simulink model "PlantModelOnHardware"  (R2018a)
settings: Solver=VariableStepAuto  StartTime=0.0  StopTime=40  RelTol=1e-3
values from neighbouring files (symbols this model uses):
  K = lqr(A,B,Qc,Rc)    [lqr_controller.m]
undefined symbols (not defined in the file or in its folder): Continuous, HIL, qc_get_step_size, Time
libraries: quarc_library x6, simulink x1, ctrlSharedLib x1
settings Model: Creator=romeo  LastModifiedBy=romeo

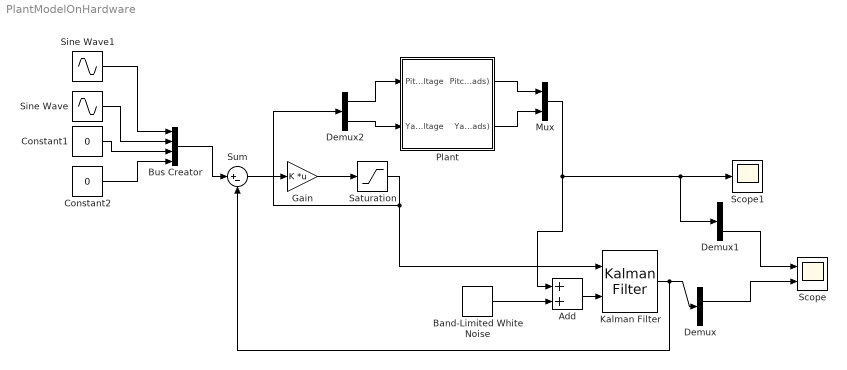
== system PlantModelOnHardware ==
  Add : Sum
  Band-Limited White Noise : simulink/Sources/Band-Limited White Noise  Cov=[0.01]  Ts=0.1  seed=[23341]
  Bus Creator : BusCreator  Inputs=4
  Constant1 : Constant  Value=0
  Constant2 : Constant  Value=0
  Demux : Demux
  Demux1 : Demux  Outputs=2
  Demux2 : Demux  Outputs=2
  Gain : Gain  Gain=K  Multiplication=Matrix(K*u)
  Kalman Filter : ctrlSharedLib/Kalman Filter  TimeDomain=Continuous-Time  UseCurrentEstimator=off  ModelSource=LTI State-Space Variable  ModelSourceVariable=sys  A=0.95  B=1  C=1  D=0  NumberOfStates=1  NumberOfInputs=1  NumberOfOutputs=1  InitialEstimateSource=Dialog  X0=0  P0=10  UseK=off  UseGH=off  NumberOfProcessNoiseInputs=1  G=1  TimeInvariantG=on  H=0  TimeInvariantH=on  Q=0.05  TimeInvariantQ=on  R=1  TimeInvariantR=on  N=0  TimeInvariantN=on  AddInputPort=on  AddEnablePort=off  OutputEstimatedY=off  OutputP=off  Ts=-1
      settings: SourceProductBaseCode=CT
  Mux : Mux  Inputs=2
  Plant : Subsystem
  Saturation : Saturate  UpperLimit=25  LowerLimit=-25
  Scope : Scope  NumInputPorts=2
  Scope1 : Scope
  Sine Wave : Sin  Amplitude=10  SampleTime=0
  Sine Wave1 : Sin  Amplitude=10  SampleTime=0
  Sum : Sum  Inputs=|+-
  wires:
  Saturation/1 -> Demux2/1, Kalman Filter/1
  Mux/1 -> Add/1, Demux1/1, Scope1/1
  Kalman Filter/1 -> Demux/1, Sum/2
  Demux1/2 -> Scope/1
  Demux/2 -> Scope/2
  Add/1 -> Kalman Filter/2
  Band-Limited White Noise/1 -> Add/2
  Sine Wave1/1 -> Bus Creator/1
  Sine Wave/1 -> Bus Creator/2
  Constant1/1 -> Bus Creator/3
  Constant2/1 -> Bus Creator/4
  Bus Creator/1 -> Sum/1
  Sum/1 -> Gain/1
  Gain/1 -> Saturation/1
  Plant/1(Pitch Position (rads)) -> Mux/1
  Plant/2(Yaw Position (rads)) -> Mux/2
  Demux2/1 -> Plant/1(Pitch Voltage)
  Demux2/2 -> Plant/2(Yaw Voltage)

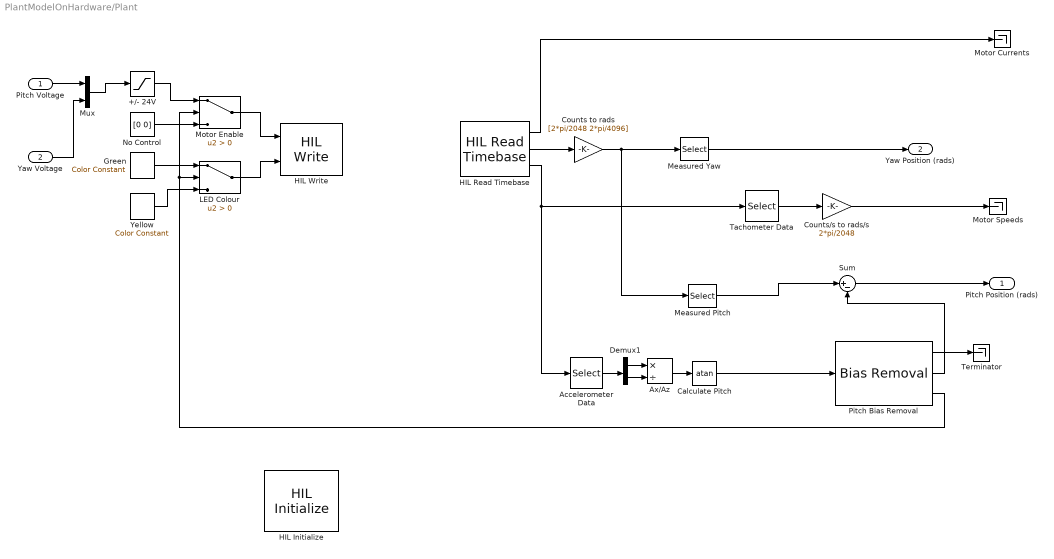
== system PlantModelOnHardware/Plant ==
  Pitch Voltage : Inport
  Yaw Voltage : Inport  Port=2
  +/- 24V : Saturate  UpperLimit=24  LowerLimit=-24
  Accelerometer Data : Selector  InputPortWidth=4  IndexOptions=Index vector (dialog)  Indices=[1 2]  OutputSizes=1
  Ax/Az : Product  Inputs=*/
  Calculate Pitch : Trigonometry  Operator=atan
  Counts to rads : Gain  Gain=[2*pi/2048 2*pi/4096]
  Counts/s to rads/s : Gain  Gain=2*pi/2048
  Demux1 : Demux  Outputs=2
  Green : quarc_library/Sources/Signals/Color Constant  color=[0 1 0]
  HIL Initialize : quarc_library/Data Acquisition/Generic/Configuration/HIL Initialize  Priority=-99  object_name=HIL-1  board_type=quanser_aero_usb  board_number=0  board_options=""  exclusive=off  active=off  hardware_clocks=[0]  clock_modes=[]  initial_clock_frequencies=[]  set_clock_params_at_start=off  set_clock_params_at_switch_in=off  set_clock_frequencies_at_start=off  set_clock_frequencies_at_switch_in=off  analog_input_channels=[0:1]  analog_input_configurations=0  analog_input_maximums=3  analog_input_minimums=-3  set_analog_input_params_at_start=off  set_analog_input_params_at_switch_in=off  analog_output_channels=[0:1]  analog_output_maximums=24  analog_output_minimums=-24  initial_analog_outputs=[0]  final_analog_outputs=[0]  watchdog_analog_outputs=[0]  set_analog_output_params_at_start=off  set_analog_output_params_at_switch_in=off  set_analog_outputs_at_start=on  set_analog_outputs_at_switch_in=off  set_analog_outputs_at_terminate=on  set_analog_outputs_at_switch_out=off  set_analog_outputs_on_watchdog=on  digital_input_channels=[]  digital_output_channels=[0:1]  digital_output_configuration=[]  initial_digital_outputs=[1]  final_digital_outputs=[0]  watchdog_digital_outputs=[0]  set_digital_output_params_at_start=off  set_digital_output_params_at_switch_in=off  set_digital_outputs_at_start=on  set_digital_outputs_at_switch_in=off  set_digital_outputs_at_terminate=on  set_digital_outputs_at_switch_out=off  set_digital_outputs_on_watchdog=on  encoder_channels=[0:3]  quadrature=[4]  encoder_filter_frequency=[]  initial_encoder_counts=[0]  set_encoder_params_at_start=off  set_encoder_params_at_switch_in=off  set_encoder_counts_at_start=on  set_encoder_counts_at_switch_in=off  pwm_channels=[]  pwm_modes=[]  pwm_frequency=[]  pwm_configuration=[]  pwm_alignment=[]  pwm_polarity=[]  pwm_leading_deadband=[]  pwm_trailing_deadband=[]  initial_pwm_outputs=[]  final_pwm_outputs=[]  watchdog_pwm_outputs=[]  set_pwm_params_at_start=off  set_pwm_params_at_switch_in=off  set_pwm_outputs_at_start=off  set_pwm_outputs_at_switch_in=off  set_pwm_outputs_at_terminate=off  set_pwm_outputs_at_switch_out=off  set_pwm_outputs_on_watchdog=off  other_output_channels=[11000:11002]  initial_other_outputs=[0 1 0]  final_other_outputs=[1 0 0]  watchdog_other_outputs=[0 0 1]  set_other_outputs_at_start=on  set_other_outputs_at_switch_in=off  set_other_outputs_at_terminate=on  set_other_outputs_at_switch_out=off  set_other_outputs_on_watchdog=on
  HIL Read Timebase : quarc_library/Data Acquisition/Generic/Timebases/HIL Read Timebase  object_name=HIL-1  clock=0  analog_channels=[0:1]  encoder_channels=[2:3]  digital_channels=[]  other_channels=[4000 4002 14000 14001]  samples_in_buffer=max(ceil(1/qc_get_step_size), 1)  active=on  vector_output=on  data_type_mode=Inherit via back propagation  encoder_data_type=double  digital_data_type=boolean
  HIL Write : quarc_library/Data Acquisition/Generic/Immediate I//O/HIL Write  object_name=HIL-1  analog_channels=[0:1]  pwm_channels=[]  digital_channels=[]  other_channels=[11000:11002]  sample_time=-1  active=off  vector_input=on
  LED Colour : Switch  Criteria=u2 > Threshold
  Measured Pitch : Selector  InputPortWidth=2  IndexOptions=Index vector (dialog)  Indices=[1]  OutputSizes=1
  Measured Yaw : Selector  InputPortWidth=2  IndexOptions=Index vector (dialog)  Indices=[2]  OutputSizes=1
  Motor Currents : Terminator
  Motor Enable : Switch  Criteria=u2 > Threshold
  Motor Speeds : Terminator
  Mux : Mux  Inputs=2
  No Control : Constant  Value=[0 0]
  Pitch Bias Removal : quarc_library/Discrete/Bias Removal  start_time=0  end_time=1  switch_id=0  sample_time=qc_get_step_size
  Sum : Sum  Inputs=|+-
  Tachometer Data : Selector  InputPortWidth=4  IndexOptions=Index vector (dialog)  Indices=[3 4]  OutputSizes=1
  Terminator : Terminator
  Yellow : quarc_library/Sources/Signals/Color Constant  color=[1 1 0]
  Pitch Position (rads) : Outport
  Yaw Position (rads) : Outport  Port=2
  wires:
  Pitch Bias Removal/3 -> Motor Enable/2, LED Colour/2
  +/- 24V/1 -> Motor Enable/1
  Motor Enable/1 -> HIL Write/1
  Green/1 -> LED Colour/1
  Yellow/1 -> LED Colour/3
  LED Colour/1 -> HIL Write/2
  No Control/1 -> Motor Enable/3
  Tachometer Data/1 -> Counts/s to rads/s/1
  Demux1/1 -> Ax/Az/1
  Demux1/2 -> Ax/Az/2
  HIL Read Timebase/2 -> Counts to rads/1
  Calculate Pitch/1 -> Pitch Bias Removal/1
  Counts/s to rads/s/1 -> Motor Speeds/1
  HIL Read Timebase/1 -> Motor Currents/1
  Accelerometer Data/1 -> Demux1/1
  HIL Read Timebase/3 -> Accelerometer Data/1, Tachometer Data/1
  Counts to rads/1 -> Measured Pitch/1, Measured Yaw/1
  Ax/Az/1 -> Calculate Pitch/1
  Pitch Bias Removal/2 -> Sum/2
  Pitch Voltage/1 -> Mux/1
  Yaw Voltage/1 -> Mux/2
  Mux/1 -> +/- 24V/1
  Pitch Bias Removal/1 -> Terminator/1
  Sum/1 -> Pitch Position (rads)/1
  Measured Pitch/1 -> Sum/1
  Measured Yaw/1 -> Yaw Position (rads)/1
